simulink model "DFIG_8_asym_voltage_dip_GSC"  (R2022b)
settings: Solver=VariableStepAuto  StartTime=0.0  StopTime=5  RelTol=1e-3
InitFcn:
  | DFIG_init8
values from neighbouring files (symbols this model uses):
  Cbus = 80e-3    (= 0.08)    [DFIG_init4.m]    (also in DFIG_init5.m; DFIG_init6.m; DFIG_init7.m; DFIG_init8.m)
  D = 1e-3    (= 0.001)    [DFIG_init1.m]    (also in DFIG_init3.m; DFIG_init4.m; DFIG_init5.m; DFIG_init6.m)
  f = 50    [DFIG_init1.m]    (also in DFIG_init3.m; DFIG_init4.m; DFIG_init5.m; DFIG_init6.m)
  fsw = 4e3    (= 4000)    [DFIG_init1.m]    (also in DFIG_init3.m; DFIG_init4.m; DFIG_init5.m; DFIG_init6.m)
  Is = 1760    [DFIG_init1.m]    (also in DFIG_init3.m; DFIG_init4.m; DFIG_init5.m; DFIG_init6.m)
  J = 127    [DFIG_init1.m]    (also in DFIG_init3.m = 63.5; DFIG_init4.m = 63.5; DFIG_init5.m; DFIG_init6.m)
  ki_id = (wni^2)*Lr*sigma    (= 491.599501999)    [DFIG_init1.m]    (also in DFIG_init3.m; DFIG_init4.m; DFIG_init5.m; DFIG_init6.m = 19.6639800799)
  ki_idg = (wnig^2)*Lg    (= 56.8489213503)    [DFIG_init4.m]    (also in DFIG_init5.m; DFIG_init6.m; DFIG_init7.m; DFIG_init8.m)
  ki_iq = ki_id    (= 491.599501999)    [DFIG_init1.m]    (also in DFIG_init3.m; DFIG_init4.m; DFIG_init5.m; DFIG_init6.m = 19.6639800799)
  ki_iqg = ki_idg    (= 56.8489213503)    [DFIG_init4.m]    (also in DFIG_init5.m; DFIG_init6.m; DFIG_init7.m; DFIG_init8.m)
  ki_n = (wnn^2)*J/p    (= 25400)    [DFIG_init1.m]    (also in DFIG_init3.m = 12700; DFIG_init4.m = 12700; DFIG_init5.m; DFIG_init6.m)
  ki_v = -300000    [DFIG_init4.m]    (also in DFIG_init5.m; DFIG_init6.m; DFIG_init7.m = -60000; DFIG_init8.m)
  Kopt = ((0.5*ro*pi* (Radio^5) *Cp_max)/(lambda_opt^3))    (= 296454.198186)    [DFIG_init3.m]    (also in DFIG_init4.m; DFIG_init5.m; DFIG_init6.m; DFIG_init7.m)
  kp_id = (2*wni*sigma*Lr)-Rr    (= 0.5771)    [DFIG_init1.m]    (also in DFIG_init3.m; DFIG_init4.m; DFIG_init5.m; DFIG_init6.m = 0.1131)
  kp_idg = (2*wnig*Lg)-Rg    (= 0.301572894745)    [DFIG_init4.m]    (also in DFIG_init5.m; DFIG_init6.m; DFIG_init7.m; DFIG_init8.m)
  kp_iq = kp_id    (= 0.5771)    [DFIG_init1.m]    (also in DFIG_init3.m; DFIG_init4.m; DFIG_init5.m; DFIG_init6.m = 0.1131)
  kp_iqg = kp_idg    (= 0.301572894745)    [DFIG_init4.m]    (also in DFIG_init5.m; DFIG_init6.m; DFIG_init7.m; DFIG_init8.m)
  kp_n = (2*wnn*J)/p    (= 2540)    [DFIG_init1.m]    (also in DFIG_init3.m = 1270; DFIG_init4.m = 1270; DFIG_init5.m; DFIG_init6.m)
  kp_v = -1000    [DFIG_init4.m]    (also in DFIG_init5.m; DFIG_init6.m; DFIG_init7.m; DFIG_init8.m)
  Kpg = 1/(1.5*Vs*sqrt(2/3))    [DFIG_init4.m]    (also in DFIG_init5.m; DFIG_init6.m; DFIG_init7.m; DFIG_init8.m)
  Kqg = -Kpg    [DFIG_init4.m]    (also in DFIG_init5.m; DFIG_init6.m; DFIG_init7.m; DFIG_init8.m)
  kT = -1.5*p*(Lm/Ls)*Fs    [DFIG_init1.m]    (also in DFIG_init3.m; DFIG_init4.m; DFIG_init5.m; DFIG_init6.m)
  Lg = 400e-6    (= 0.0004)    [DFIG_init4.m]    (also in DFIG_init5.m; DFIG_init6.m; DFIG_init7.m; DFIG_init8.m)
  Lr = Lm + Lsi    (= 0.002587)    [DFIG_init1.m]    (also in DFIG_init3.m; DFIG_init4.m; DFIG_init5.m; DFIG_init6.m)
  Lsi = 0.087e-3    (= 8.7e-05)    [DFIG_init1.m]    (also in DFIG_init3.m; DFIG_init4.m; DFIG_init5.m; DFIG_init6.m)
  N = 100    [DFIG_init3.m]    (also in DFIG_init4.m; DFIG_init5.m; DFIG_init6.m; DFIG_init7.m)
  p = 2    [DFIG_init1.m]    (also in DFIG_init3.m; DFIG_init4.m; DFIG_init5.m; DFIG_init6.m)
  Ps = 2e6    (= 2000000)    [DFIG_init1.m]    (also in DFIG_init3.m; DFIG_init4.m; DFIG_init5.m; DFIG_init6.m)
  Radio = 42    [DFIG_init3.m]    (also in DFIG_init4.m; DFIG_init5.m; DFIG_init6.m; DFIG_init7.m)
  Rcrowbar = 0.2    [DFIG_init5.m]    (also in DFIG_init6.m; DFIG_init7.m; DFIG_init8.m; DFIG_init9.m)
  Rg = 20e-6    (= 2e-05)    [DFIG_init4.m]    (also in DFIG_init5.m; DFIG_init6.m; DFIG_init7.m; DFIG_init8.m)
  ro = 1.225    [DFIG_init3.m]    (also in DFIG_init4.m; DFIG_init5.m; DFIG_init6.m; DFIG_init7.m)
  Rr = 2.9e-3    (= 0.0029)    [DFIG_init1.m]    (also in DFIG_init3.m; DFIG_init4.m; DFIG_init5.m; DFIG_init6.m)
  Rs = 2.6e-3    (= 0.0026)    [DFIG_init1.m]    (also in DFIG_init3.m; DFIG_init4.m; DFIG_init5.m; DFIG_init6.m)
  sigma = 1-Lm^2/(Ls*Lr)    (= 0.0661284179513)    [DFIG_init1.m]    (also in DFIG_init3.m; DFIG_init4.m; DFIG_init5.m; DFIG_init6.m)
  smax = 1/3    (= 0.333333333333)    [DFIG_init1.m]    (also in DFIG_init3.m; DFIG_init4.m; DFIG_init5.m; DFIG_init6.m)
  t_dip = 3    [DFIG_init5.m]    (also in DFIG_init6.m = 30; DFIG_init7.m; DFIG_init8.m; DFIG_init9.m)
  t_normal = 4.17    [DFIG_init5.m]    (also in DFIG_init6.m = 417; DFIG_init7.m = 4.2; DFIG_init8.m = 4.2; DFIG_init9.m)
  t_recover = 3.5    [DFIG_init5.m]    (also in DFIG_init6.m = 35; DFIG_init7.m; DFIG_init8.m; DFIG_init9.m)
  tab_lambda = [0.1:0.01:11.8]    [DFIG_init3.m]    (also in DFIG_init4.m; DFIG_init5.m; DFIG_init6.m; DFIG_init7.m)
  Tcrowbar = 0.1    [DFIG_init5.m]    (also in DFIG_init6.m; DFIG_init7.m; DFIG_init8.m; DFIG_init9.m)
  Tem = 12732    [DFIG_init1.m]    (also in DFIG_init3.m; DFIG_init4.m; DFIG_init5.m; DFIG_init6.m)
  Ts = 1/fsw/50    (= 5e-06)    [DFIG_init1.m]    (also in DFIG_init3.m; DFIG_init4.m; DFIG_init5.m; DFIG_init6.m)
  Vbus = Vr_stator*sqrt(2)    [DFIG_init1.m]    (also in DFIG_init3.m; DFIG_init4.m = 1150; DFIG_init5.m = 1150; DFIG_init6.m = 1150)
  Vs = 690    [DFIG_init1.m]    (also in DFIG_init3.m; DFIG_init4.m; DFIG_init5.m; DFIG_init6.m)
undefined symbols (not defined in the file or in its folder): Ct, DiscIntNeverNeededParam
libraries: spsSeriesRLCBranchLib x5, spsSecondOrderFilterLib x4, spsUniversalBridgeLib x3, spsThreePhaseVIMeasurementLib x3, spsPLL3phLib x2, spsPWMGenerator2LevelLib x2, spsAsynchronousMachineSIUnitsLib x1, spsGroundLib x1, spsIdealSwitchLib x1, spsThreePhaseProgrammableVoltageSourceLib x1, spsThreePhaseTransformerTwoWindingsLib x1, spsEdgeDetectorLib x1
settings Model: SimulationMode=accelerator  Creator=Qingyuan  LastModifiedBy=Qingyuan

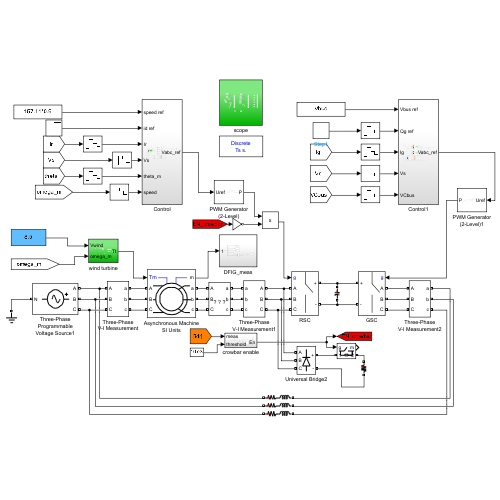
[thumbnail: Simulink's stored preview of the top-level diagram]
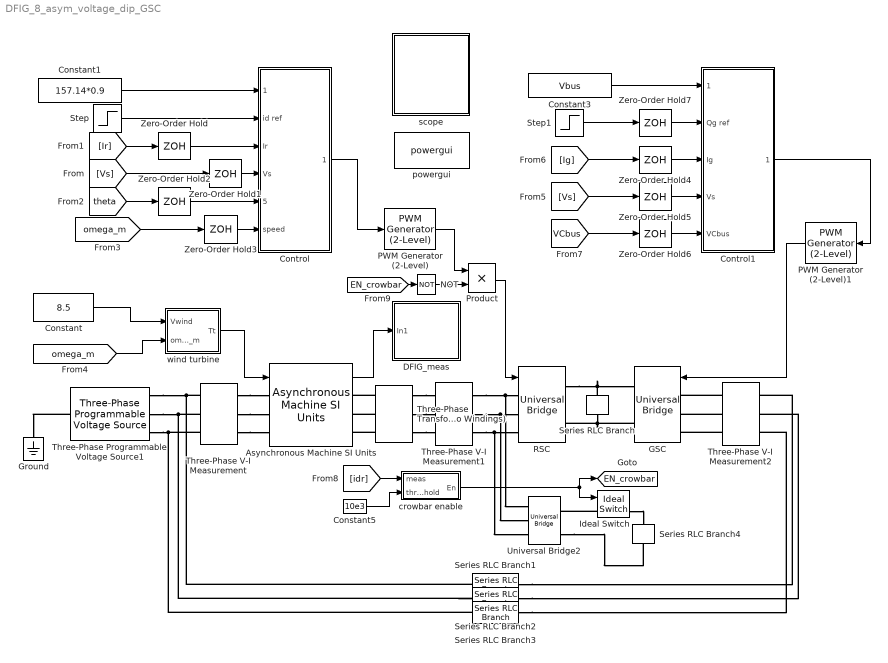
== system DFIG_8_asym_voltage_dip_GSC ==
  Asynchronous Machine SI Units : spsAsynchronousMachineSIUnitsLib/Asynchronous Machine SI Units  RotorType=Wound  PresetModel=No  MechanicalLoad=Torque Tm  ShowDetailedParameters=on  ReferenceFrame=Rotor  Units=SI  MeasurementBus=off  NominalParameters=[Ps Vs f]  VoltageRatio=1  Stator=[Rs Lsi]  Rotor=[Rr Lsi]  Cage1=[0.4155 0.002066]  Cage2=[0.4168 0.0003495]  Lm=Lm  Mechanical=[J D p]  PolePairs=2  InitialConditions=[1 0 0 0 0 0 0 0]  SimulateSaturation=off  Saturation=[14.03593122, 27.81365428, 53.79336849, 72.68890987, 97.98006896, 148.6815601, 215.7428561, 302.9841135, 428.7778367 ; 230, 322, 414, 460, 506, 552, 598, 644, 690]  LoadFlowParameters=1492000  TsPowergui=0  TsBlock=-1  IterativeModel=Trapezoidal non iterative  IterativeDiscreteModel=Trapezoidal non iterative  Pmec=1.4e6
  Constant : Constant  Value=8.5
  Constant1 : Constant  Value=157.14*0.9
  Constant3 : Constant  Value=Vbus
  Constant5 : Constant  Value=10e3
  Control : Subsystem
  Control1 : Subsystem
  DFIG_meas : Subsystem
  GSC : spsUniversalBridgeLib/Universal Bridge  Arms=3  SnubberResistance=1e5  SnubberCapacitance=inf  Device=Ideal Switches  Ron=1e-3  Lon=0  ForwardVoltages="[  0  0  ]"  ForwardVoltage=0  GTOparameters=[ 10e-6 , 20e-6 ]  IGBTparameters=[ 1e-6 , 2e-6 ]  Measurements=None  Measurements_2=None  converterType=Rectifier
  Ground : spsGroundLib/Ground  LConnTagsString=a
  Ideal Switch : spsIdealSwitchLib/Ideal Switch  Ron=0.001  Lon=0  IC=0  Rs=1e5  Cs=inf  Measurements=on
  NOT : Logic  Operator=NOT  IconShape=distinctive  AllPortsSameDT=off  OutDataTypeStr=boolean
  PWM Generator (2-Level) : spsPWMGenerator2LevelLib/PWM Generator (2-Level)  ModulatorType=Three-phase bridge (6 pulses)  ModulatorMode=Unsynchronized  Fc=fsw  Pc=0  nF=27  MinMax="[ -1  1 ]"  SamplingTechnique=Symmetrical regular (single edge)  ModulatingSignals=off  m=0.8  Freq=60  Phase=0  Ts=0  ShowCarrierOutport=off
  PWM Generator (2-Level)1 : spsPWMGenerator2LevelLib/PWM Generator (2-Level)  ModulatorType=Three-phase bridge (6 pulses)  ModulatorMode=Unsynchronized  Fc=fsw  Pc=0  nF=27  MinMax="[ -1  1 ]"  SamplingTechnique=Symmetrical regular (single edge)  ModulatingSignals=off  m=0.8  Freq=60  Phase=0  Ts=0  ShowCarrierOutport=off
  Product : Product
  RSC : spsUniversalBridgeLib/Universal Bridge  Arms=3  SnubberResistance=1e5  SnubberCapacitance=inf  Device=Ideal Switches  Ron=1e-3  Lon=0  ForwardVoltages="[  0  0  ]"  ForwardVoltage=0  GTOparameters=[ 10e-6 , 20e-6 ]  IGBTparameters=[ 1e-6 , 2e-6 ]  Measurements=None  Measurements_2=None  converterType=Rectifier
  Series RLC Branch : spsSeriesRLCBranchLib/Series RLC Branch  LConnTagsString=__new0  RConnTagsString=__new0  BranchType=C  Resistance=1  Inductance=1e-3  SetiL0=off  InitialCurrent=0  Capacitance=Cbus  Setx0=off  InitialVoltage=0  Measurements=Branch voltage
  Series RLC Branch1 : spsSeriesRLCBranchLib/Series RLC Branch  LConnTagsString=__new0  RConnTagsString=__new0  BranchType=RL  Resistance=Rg  Inductance=Lg  SetiL0=off  InitialCurrent=0  Capacitance=1e-6  Setx0=off  InitialVoltage=0  Measurements=None
  Series RLC Branch2 : spsSeriesRLCBranchLib/Series RLC Branch  LConnTagsString=__new0  RConnTagsString=__new0  BranchType=RL  Resistance=Rg  Inductance=Lg  SetiL0=off  InitialCurrent=0  Capacitance=1e-6  Setx0=off  InitialVoltage=0  Measurements=None
  Series RLC Branch3 : spsSeriesRLCBranchLib/Series RLC Branch  LConnTagsString=__new0  RConnTagsString=__new0  BranchType=RL  Resistance=Rg  Inductance=Lg  SetiL0=off  InitialCurrent=0  Capacitance=1e-6  Setx0=off  InitialVoltage=0  Measurements=None
  Series RLC Branch4 : spsSeriesRLCBranchLib/Series RLC Branch  LConnTagsString=__new0  RConnTagsString=__new0  BranchType=R  Resistance=Rcrowbar  Inductance=1e-3  SetiL0=off  InitialCurrent=0  Capacitance=Cbus  Setx0=off  InitialVoltage=0  Measurements=Branch current
  Step : Step  Time=t_dip+0.1  After=0.25*Is  SampleTime=0
  Step1 : Step  Time=t_dip+0.1  After=-500e3  SampleTime=0
  Three-Phase Programmable Voltage Source1 : spsThreePhaseProgrammableVoltageSourceLib/Three-Phase Programmable Voltage Source  PositiveSequence=[Vs 0 f]  VariationEntity=None  VariationType=Ramp  VariationTypeAlt=Step  VariationStep=0.5  VariationRate=15  VariationMagnitude=0.3  VariationFrequency=2  VariationTiming=[t_recover t_normal]  VariationPhaseA=off  Amplitudes=[1 0.8 1.2 1.0]  TimeValues=[0 0.1 0.15 0.2]  HarmonicGeneration=on  HarmonicA=[1 0.3 180 1]  HarmonicB=[1 0.2 0 2]  Timing="[t_dip  t_normal]"  BusType=swing  Pref=0  Qref=0  Qmin=-inf  Qmax=inf
  Three-Phase Transformer (Two Windings) : spsThreePhaseTransformerTwoWindingsLib/Three-Phase Transformer (Two Windings)  Winding1Connection=Y  Winding2Connection=Y  CoreType=Three single-phase transformers  SetSaturation=off  Hysteresis=off  DataFile='hysteresis'  SetInitialFlux=off  Measurements=None  UNITS=SI  NominalPower=[ Ps , f ]  Winding1=[Vs 0 0]  Winding2=[Vs/u 0 0]  Rm=1.3506e+08  Lm=4.299e+05  L0=0.5  Saturation=[0 0;0.0053322 2292.3;2.2218 2903.6]  InitialFluxes=[ 0.8 , -0.8 , 0.7 ]  BreakLoop=off  DiscreteSolver=Trapezoidal iterative  DataType=on  TransfoNumber=1
  Three-Phase V-I Measurement : spsThreePhaseVIMeasurementLib/Three-Phase V-I Measurement  VoltageMeasurement=phase-to-ground  SetLabelV=on  LabelV=Vs  Vpu=off  VpuLL=off  CurrentMeasurement=yes  SetLabelI=on  LabelI=Is  Ipu=off  Pbase=100e6  Vbase=500e3  OutputType=Complex  PhasorSimulation=off  PSBequivalent=0
  Three-Phase V-I Measurement1 : spsThreePhaseVIMeasurementLib/Three-Phase V-I Measurement  VoltageMeasurement=no  SetLabelV=off  LabelV=Vc  Vpu=off  VpuLL=off  CurrentMeasurement=yes  SetLabelI=on  LabelI=Ir  Ipu=off  Pbase=100e6  Vbase=500e3  OutputType=Complex  PhasorSimulation=off  PSBequivalent=0
  Three-Phase V-I Measurement2 : spsThreePhaseVIMeasurementLib/Three-Phase V-I Measurement  VoltageMeasurement=no  SetLabelV=off  LabelV=Vc  Vpu=off  VpuLL=off  CurrentMeasurement=yes  SetLabelI=on  LabelI=Ig  Ipu=off  Pbase=100e6  Vbase=500e3  OutputType=Complex  PhasorSimulation=off  PSBequivalent=0
  Universal Bridge2 : spsUniversalBridgeLib/Universal Bridge  Arms=3  SnubberResistance=1e5  SnubberCapacitance=inf  Device=Diodes  Ron=1e-3  Lon=0  ForwardVoltages="[  0  0  ]"  ForwardVoltage=0  GTOparameters=[ 10e-6 , 20e-6 ]  IGBTparameters=[ 1e-6 , 2e-6 ]  Measurements=None  Measurements_2=None  converterType=Rectifier
  Zero-Order Hold{,1..7} (8 alike) : ZeroOrderHold  SampleTime=1/fsw
  crowbar enable : Subsystem
  powergui : spspowerguiLib/powergui  Priority=1  SimulationMode=Discrete  SampleTime=Ts  frequency=60  Iterations=50  frequencyindice=50  Pbase=100e6  ErrMax=1e-4  UnitsV=kV  UnitsW=MW  buscounter=0  FunctionMessages=off  echomessages=off  EnableUseOfTLC=off  CurrentSourceSwitches=off  DisableSnubberDevices=off  DisableRonSwitches=off  DisableVfSwitches=off  DisplayEquations=off  AutomaticDiscreteSolvers=off  SolverType=Tustin/Backward Euler (TBE)  Interpol=off  ExternalGateDelay=off  methode=off  Ts=100  x0status=blocks  SPID=on  SwTol=0  HookPort=off  NonlinearTolerance=1e-4  nMaxIteration=100  ContinueOnMaxIteration=off  RestoreLinks=warning  ResistiveCurrentMeasurement=off  Frange=[0:2:500]  Ylog=off  Xlog=on  ShowGrid=off  save=off  variable=ZData  structure=0  ZoomFFT=off  StartTime=0.0  cycles=1  DisplayStyle=1  fundamental=60  FreqAxis=off  MaxFrequency=1000  frequencyindicesteady=1  RmsSteady=1  display=off
  scope : Subsystem
  wind turbine : Subsystem
  tag scope: EN_crowbar=global
  wires:
  Control/1(Vabc_ref) -> PWM Generator (2-Level)/1
  [Vs] -> Zero-Order Hold1/1
  [Ir] -> Zero-Order Hold/1
  Constant1/1 -> Control/1(speed ref)
  Step/1 -> Control/2(id ref)
  [theta] -> Zero-Order Hold2/1
  [omega_m] -> Zero-Order Hold3/1
  Asynchronous Machine SI Units/1 -> DFIG_meas/1(In1)
  Zero-Order Hold/1 -> Control/3(Ir)
  Zero-Order Hold1/1 -> Control/4(Vs)
  Zero-Order Hold2/1 -> Control/5(theta_m)
  Zero-Order Hold3/1 -> Control/6(speed)
  Constant/1 -> wind turbine/1(Vwind)
  wind turbine/1(Tt) -> Asynchronous Machine SI Units/1
  [omega_m] -> wind turbine/2(omega_m)
  Zero-Order Hold5/1 -> Control1/4(Vs)
  Zero-Order Hold4/1 -> Control1/3(Ig)
  Constant3/1 -> Control1/1(Vbus ref)
  [Ig] -> Zero-Order Hold4/1
  [Vs] -> Zero-Order Hold5/1
  Control1/1(Vabc_ref) -> PWM Generator (2-Level)1/1
  [VCbus] -> Zero-Order Hold6/1
  Zero-Order Hold6/1 -> Control1/5(VCbus)
  Zero-Order Hold7/1 -> Control1/2(Qg ref)
  Constant5/1 -> crowbar enable/2(threshold)
  crowbar enable/1(En) -> Ideal Switch/1, [EN_crowbar]
  [idr] -> crowbar enable/1(meas)
  NOT/1 -> Product/2
  [EN_crowbar] -> NOT/1
  PWM Generator (2-Level)1/1 -> GSC/1
  PWM Generator (2-Level)/1 -> Product/1
  Product/1 -> RSC/1
  Step1/1 -> Zero-Order Hold7/1
  connections:
  Three-Phase Programmable Voltage Source1/LConn1 -- Ground/LConn1
  Three-Phase V-I Measurement/LConn1 -- Three-Phase Programmable Voltage Source1/RConn1 -- Series RLC Branch1/LConn1
  Three-Phase V-I Measurement/LConn2 -- Three-Phase Programmable Voltage Source1/RConn2 -- Series RLC Branch2/LConn1
  Three-Phase V-I Measurement/LConn3 -- Series RLC Branch3/LConn1 -- Three-Phase Programmable Voltage Source1/RConn3
  Three-Phase V-I Measurement/RConn1 -- Asynchronous Machine SI Units/LConn1
  Three-Phase V-I Measurement/RConn2 -- Asynchronous Machine SI Units/LConn2
  Three-Phase V-I Measurement/RConn3 -- Asynchronous Machine SI Units/LConn3
  Three-Phase V-I Measurement1/LConn1 -- Universal Bridge2/LConn1 -- RSC/LConn1
  Three-Phase V-I Measurement1/LConn3 -- Universal Bridge2/LConn3 -- RSC/LConn3
  Three-Phase V-I Measurement1/LConn2 -- Universal Bridge2/LConn2 -- RSC/LConn2
  Three-Phase Transformer (Two Windings)/RConn1 -- Three-Phase V-I Measurement1/RConn1
  Three-Phase Transformer (Two Windings)/RConn2 -- Three-Phase V-I Measurement1/RConn2
  Three-Phase Transformer (Two Windings)/RConn3 -- Three-Phase V-I Measurement1/RConn3
  RSC/RConn1 -- Series RLC Branch/LConn1 -- GSC/RConn1
  GSC/RConn2 -- RSC/RConn2 -- Series RLC Branch/RConn1
  Three-Phase V-I Measurement2/LConn1 -- GSC/LConn1
  Three-Phase V-I Measurement2/LConn2 -- GSC/LConn2
  Three-Phase V-I Measurement2/LConn3 -- GSC/LConn3
  Series RLC Branch1/RConn1 -- Three-Phase V-I Measurement2/RConn1
  Series RLC Branch2/RConn1 -- Three-Phase V-I Measurement2/RConn2
  Series RLC Branch3/RConn1 -- Three-Phase V-I Measurement2/RConn3
  Three-Phase Transformer (Two Windings)/LConn3 -- Asynchronous Machine SI Units/RConn3
  Three-Phase Transformer (Two Windings)/LConn2 -- Asynchronous Machine SI Units/RConn2
  Three-Phase Transformer (Two Windings)/LConn1 -- Asynchronous Machine SI Units/RConn1
  Ideal Switch/LConn1 -- Universal Bridge2/RConn1
  Ideal Switch/RConn1 -- Series RLC Branch4/LConn1
  Universal Bridge2/RConn2 -- Series RLC Branch4/RConn1

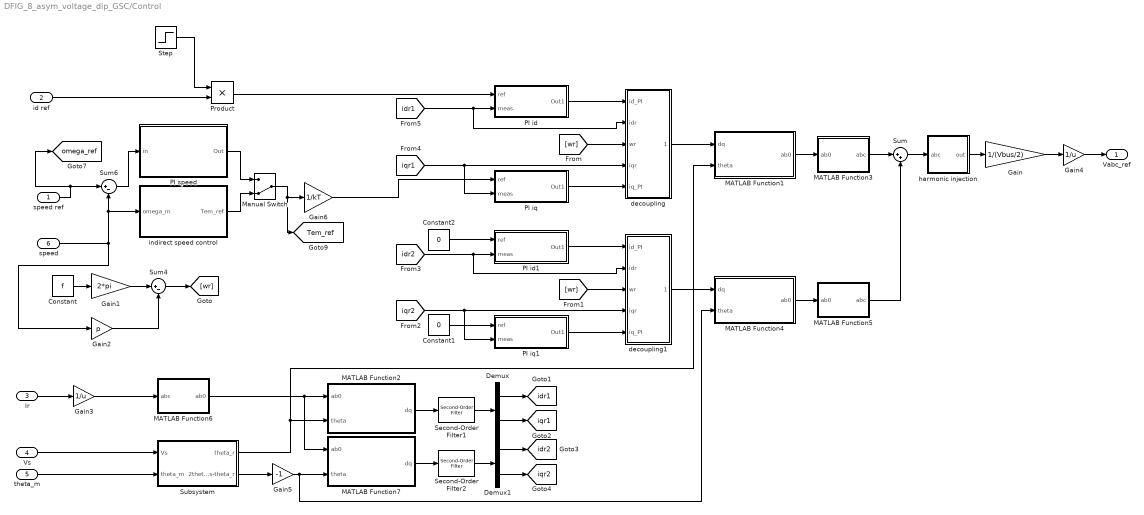
== system DFIG_8_asym_voltage_dip_GSC/Control ==
  speed ref : Inport
  id ref : Inport  Port=2
  Ir : Inport  Port=3
  Vs : Inport  Port=4
  theta_m : Inport  Port=5
  speed : Inport  Port=6
  Constant : Constant  Value=f
  Constant1 : Constant  Value=0
  Constant2 : Constant  Value=0
  Demux : Demux  Outputs=2
  Demux1 : Demux  Outputs=2
  Gain : Gain  Gain=1/(Vbus/2)
  Gain1 : Gain  Gain=2*pi
  Gain2 : Gain  Gain=p
  Gain3 : Gain  Gain=1/u
  Gain4 : Gain  Gain=1/u
  Gain5 : Gain  Gain=-1
  Gain6 : Gain  Gain=1/kT
  MATLAB Function1 : MATLAB Function  TreatAsAtomicUnit=on
  MATLAB Function2 : MATLAB Function  TreatAsAtomicUnit=on
  MATLAB Function3 : MATLAB Function  TreatAsAtomicUnit=on
  MATLAB Function4 : MATLAB Function  TreatAsAtomicUnit=on
  MATLAB Function5 : MATLAB Function  TreatAsAtomicUnit=on
  MATLAB Function6 : MATLAB Function  TreatAsAtomicUnit=on
  MATLAB Function7 : MATLAB Function  TreatAsAtomicUnit=on
  Manual Switch : ManualSwitch  CurrentSetting=0
  PI id : Subsystem
  PI id1 : Subsystem
  PI iq : Subsystem
  PI iq1 : Subsystem
  PI speed : Subsystem
  Product : Product
  Second-Order Filter1 : spsSecondOrderFilterLib/Second-Order Filter  FilterType=Bandstop (Notch)  Fo=100  Zeta=0.707  Ts=0  Initialize=on  Vac_Init="[0,  0,  50]"  Vdc_Init=0  PlotResponse=off  FreqRange=[0, 500, 1]
      settings: LibrarySourceBlock=|
      | sps_lib/Control/Filters/Second-Order
      | Filter
  Second-Order Filter2 : spsSecondOrderFilterLib/Second-Order Filter  FilterType=Bandstop (Notch)  Fo=100  Zeta=0.707  Ts=0  Initialize=on  Vac_Init="[0,  0,  50]"  Vdc_Init=0  PlotResponse=off  FreqRange=[0, 500, 1]
      settings: LibrarySourceBlock=|
      | sps_lib/Control/Filters/Second-Order
      | Filter
  Step : Step  Time=t_normal+1  Before=1  After=0  SampleTime=0
  Subsystem : Subsystem
  Sum : Sum  Inputs=|++
  Sum4 : Sum  Inputs=|+-
  Sum6 : Sum  Inputs=|+-
  decoupling : Subsystem
  decoupling1 : Subsystem
  harmonic injection : Subsystem
  indirect speed control : Subsystem
  Vabc_ref : Outport
  tag scope: Tem_ref=global, idr1=global, idr2=global, iqr1=global, iqr2=global, omega_ref=global
  wires:
  MATLAB Function1/1(ab0) -> MATLAB Function3/1(ab0)
  Gain/1 -> Gain4/1
  harmonic injection/1(out) -> Gain/1
  Vs/1 -> Subsystem/1(Vs)
  theta_m/1 -> Subsystem/2(theta_m)
  MATLAB Function6/1(ab0) -> MATLAB Function7/1(ab0), MATLAB Function2/1(ab0)
  Ir/1 -> Gain3/1
  Subsystem/1(theta_r) -> MATLAB Function2/2(theta), MATLAB Function1/2(theta)
  Constant/1 -> Gain1/1
  Gain1/1 -> Sum4/1
  Gain2/1 -> Sum4/2
  Sum4/1 -> [wr]
  MATLAB Function2/1(dq) -> Second-Order Filter1/1
  Demux/2 -> [iqr1]
  Demux/1 -> [idr1]
  Sum6/1 -> PI speed/1(in)
  speed ref/1 -> [omega_ref], Sum6/1
  [idr1] -> decoupling/2(idr), PI id/2(meas)
  [iqr1] -> PI iq/2(meas), decoupling/4(iqr)
  Manual Switch/1 -> [Tem_ref], Gain6/1
  PI speed/1(Out) -> Manual Switch/1
  indirect speed control/1(Tem_ref) -> Manual Switch/2
  speed/1 -> Gain2/1, indirect speed control/1(omega_m), Sum6/2
  Gain3/1 -> MATLAB Function6/1(abc)
  Gain4/1 -> Vabc_ref/1
  id ref/1 -> Product/2
  Step/1 -> Product/1
  [wr] -> decoupling/3(wr)
  decoupling/1(Vref_dq) -> MATLAB Function1/1(dq)
  Product/1 -> PI id/1(ref)
  PI id/1(Out1) -> decoupling/1(id_PI)
  Gain6/1 -> PI iq/1(ref)
  PI iq/1(Out1) -> decoupling/5(iq_PI)
  PI iq1/1(Out1) -> decoupling1/5(iq_PI)
  PI id1/1(Out1) -> decoupling1/1(id_PI)
  decoupling1/1(Vref_dq) -> MATLAB Function4/1(dq)
  [wr] -> decoupling1/3(wr)
  [iqr2] -> decoupling1/4(iqr), PI iq1/2(meas)
  [idr2] -> PI id1/2(meas), decoupling1/2(idr)
  MATLAB Function4/1(ab0) -> MATLAB Function5/1(ab0)
  Constant1/1 -> PI iq1/1(ref)
  Constant2/1 -> PI id1/1(ref)
  MATLAB Function3/1(abc) -> Sum/1
  Sum/1 -> harmonic injection/1(abc)
  MATLAB Function5/1(abc) -> Sum/2
  Subsystem/2(2theta_s-theta_r) -> Gain5/1
  Gain5/1 -> MATLAB Function4/2(theta), MATLAB Function7/2(theta)
  Demux1/1 -> [idr2]
  Demux1/2 -> [iqr2]
  MATLAB Function7/1(dq) -> Second-Order Filter2/1
  Second-Order Filter1/1 -> Demux/1
  Second-Order Filter2/1 -> Demux1/1

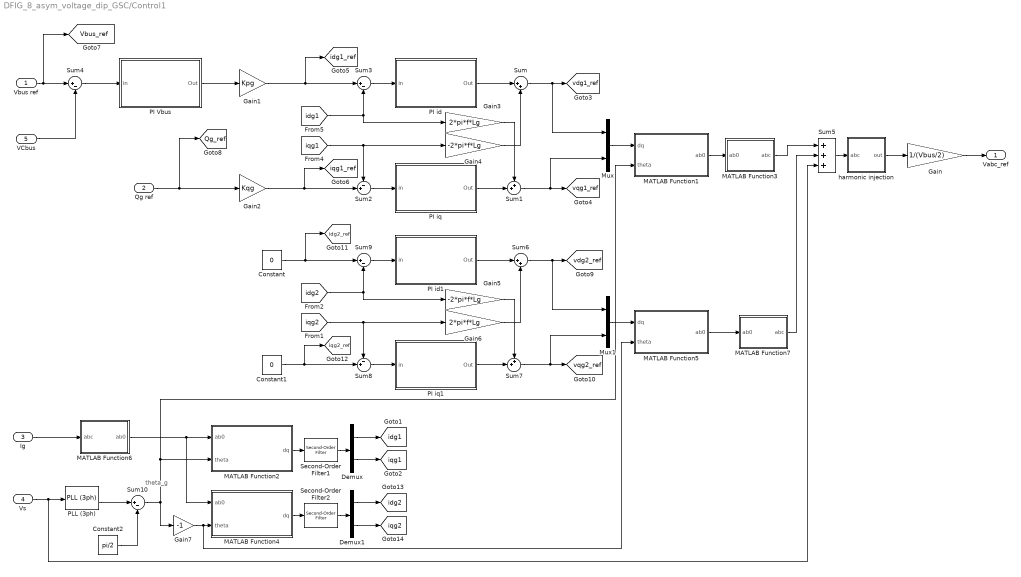
== system DFIG_8_asym_voltage_dip_GSC/Control1 ==
  note: theta_g
  Vbus ref : Inport
  Qg ref : Inport  Port=2
  Ig : Inport  Port=3
  Vs : Inport  Port=4
  VCbus : Inport  Port=5
  Constant : Constant  Value=0
  Constant1 : Constant  Value=0
  Constant2 : Constant  Value=pi/2
  Demux : Demux  Outputs=2
  Demux1 : Demux  Outputs=2
  Gain : Gain  Gain=1/(Vbus/2)
  Gain1 : Gain  Gain=Kpg
  Gain2 : Gain  Gain=Kqg
  Gain3 : Gain  Gain=2*pi*f*Lg
  Gain4 : Gain  Gain=-2*pi*f*Lg
  Gain5 : Gain  Gain=-2*pi*f*Lg
  Gain6 : Gain  Gain=2*pi*f*Lg
  Gain7 : Gain  Gain=-1
  MATLAB Function1 : MATLAB Function  TreatAsAtomicUnit=on
  MATLAB Function2 : MATLAB Function  TreatAsAtomicUnit=on
  MATLAB Function3 : MATLAB Function  TreatAsAtomicUnit=on
  MATLAB Function4 : MATLAB Function  TreatAsAtomicUnit=on
  MATLAB Function5 : MATLAB Function  TreatAsAtomicUnit=on
  MATLAB Function6 : MATLAB Function  TreatAsAtomicUnit=on
  MATLAB Function7 : MATLAB Function  TreatAsAtomicUnit=on
  Mux : Mux  Inputs=2
  Mux1 : Mux  Inputs=2
  PI Vbus : Subsystem
  PI id : Subsystem
  PI id1 : Subsystem
  PI iq : Subsystem
  PI iq1 : Subsystem
  PLL (3ph) : spsPLL3phLib/PLL (3ph)  Fmin=45  Par_Init=[0, 50]  ParK=[180, 3200, 1]  TcD=0.01  MaxRateChangeFreq=12  FilterCutOffFreq=25  Ts=1/fsw  AGC=on
  Second-Order Filter1 : spsSecondOrderFilterLib/Second-Order Filter  FilterType=Bandstop (Notch)  Fo=100  Zeta=0.707  Ts=0  Initialize=on  Vac_Init="[0,  0,  50]"  Vdc_Init=0  PlotResponse=off  FreqRange=[0, 500, 1]
      settings: LibrarySourceBlock=|
      | sps_lib/Control/Filters/Second-Order
      | Filter
  Second-Order Filter2 : spsSecondOrderFilterLib/Second-Order Filter  FilterType=Bandstop (Notch)  Fo=100  Zeta=0.707  Ts=0  Initialize=on  Vac_Init="[0,  0,  50]"  Vdc_Init=0  PlotResponse=off  FreqRange=[0, 500, 1]
      settings: LibrarySourceBlock=|
      | sps_lib/Control/Filters/Second-Order
      | Filter
  Sum : Sum  Inputs=|++
  Sum1 : Sum  Inputs=++|
  Sum{3..4,9..10} (4 alike) : Sum  Inputs=|+-
  Sum2 : Sum  Inputs=-+|
  Sum5 : Sum  Inputs=+++
  Sum6 : Sum  Inputs=|++
  Sum7 : Sum  Inputs=++|
  Sum8 : Sum  Inputs=-+|
  harmonic injection : Subsystem
  Vabc_ref : Outport
  tag scope: Qg_ref=global, Vbus_ref=global, idg1=global, idg1_ref=global, idg2=global, idg2_ref=global, iqg1=global, iqg1_ref=global, iqg2=global, iqg2_ref=global, vdg1_ref=global, vdg2_ref=global, vqg1_ref=global, vqg2_ref=global
  wires:
  PI Vbus/1(Out) -> Gain1/1
  [iqg1] -> Sum2/1, Gain4/1
  Gain3/1 -> Sum1/1
  PI iq/1(Out) -> Sum1/2
  Gain4/1 -> Sum/2
  PI id/1(Out) -> Sum/1
  [idg1] -> Gain3/1, Sum3/2
  Gain2/1 -> Sum2/2, [iqg1_ref]
  Mux/1 -> MATLAB Function1/1(dq)
  Sum1/1 -> Mux/2, [vqg1_ref]
  Sum/1 -> [vdg1_ref], Mux/1
  Demux/1 -> [idg1]
  Demux/2 -> [iqg1]
  MATLAB Function2/1(dq) -> Second-Order Filter1/1
  Sum3/1 -> PI id/1(in)
  Sum2/1 -> PI iq/1(in)
  Ig/1 -> MATLAB Function6/1(abc)
  MATLAB Function6/1(ab0) -> MATLAB Function4/1(ab0), MATLAB Function2/1(ab0)
  harmonic injection/1(out) -> Gain/1
  Gain/1 -> Vabc_ref/1
  MATLAB Function1/1(ab0) -> MATLAB Function3/1(ab0)
  Gain1/1 -> [idg1_ref], Sum3/1
  Qg ref/1 -> [Qg_ref], Gain2/1
  VCbus/1 -> Sum4/2
  Vbus ref/1 -> [Vbus_ref], Sum4/1
  Sum4/1 -> PI Vbus/1(in)
  Sum5/1 -> harmonic injection/1(abc)
  MATLAB Function3/1(abc) -> Sum5/1
  Constant/1 -> [idg2_ref], Sum9/1
  MATLAB Function5/1(ab0) -> MATLAB Function7/1(ab0)
  Sum8/1 -> PI iq1/1(in)
  Sum9/1 -> PI id1/1(in)
  Sum6/1 -> Mux1/1, [vdg2_ref]
  Sum7/1 -> [vqg2_ref], Mux1/2
  Mux1/1 -> MATLAB Function5/1(dq)
  Constant1/1 -> [iqg2_ref], Sum8/2
  [idg2] -> Sum9/2, Gain5/1
  PI id1/1(Out) -> Sum6/1
  Gain6/1 -> Sum6/2
  PI iq1/1(Out) -> Sum7/2
  Gain5/1 -> Sum7/1
  [iqg2] -> Gain6/1, Sum8/1
  Constant2/1 -> Sum10/2
  PLL (3ph)/2 -> Sum10/1
  Vs/1 -> Sum5/3, PLL (3ph)/1
  Second-Order Filter1/1 -> Demux/1
  Sum10/1 -> Gain7/1, MATLAB Function2/2(theta), MATLAB Function1/2(theta)
  Second-Order Filter2/1 -> Demux1/1
  MATLAB Function4/1(dq) -> Second-Order Filter2/1
  Demux1/2 -> [iqg2]
  Demux1/1 -> [idg2]
  Gain7/1 -> MATLAB Function5/2(theta), MATLAB Function4/2(theta)
  MATLAB Function7/1(abc) -> Sum5/2

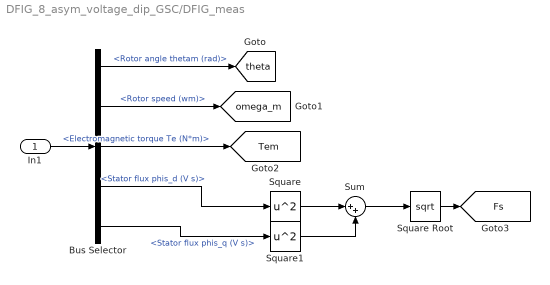
== system DFIG_8_asym_voltage_dip_GSC/DFIG_meas ==
  In1 : Inport
  Bus Selector : BusSelector  OutputSignals=Mechanical.Rotor angle thetam (rad),Mechanical.Rotor speed (wm),Mechanical.Electromagnetic torque Te (N*m),Stator measurements.Stator flux phis_d (V s),Stator measurements.Stator flux phis_q (V s)
  Square : Math  Operator=square
  Square Root : Sqrt
  Square1 : Math  Operator=square
  Sum : Sum  Inputs=|++
  tag scope: Fs=global, Tem=global, omega_m=global, theta=global
  wires:
  Bus Selector/1 -> [theta]  "<Rotor angle thetam (rad)>"
  Bus Selector/2 -> [omega_m]  "<Rotor speed (wm)>"
  In1/1 -> Bus Selector/1
  Bus Selector/3 -> [Tem]  "<Electromagnetic torque Te (N*m)>"
  Bus Selector/4 -> Square/1  "<Stator flux phis_d (V s)>"
  Bus Selector/5 -> Square1/1  "<Stator flux phis_q (V s)>"
  Square/1 -> Sum/1
  Sum/1 -> Square Root/1
  Square1/1 -> Sum/2
  Square Root/1 -> [Fs]

== system DFIG_8_asym_voltage_dip_GSC/crowbar enable ==
  meas : Inport
  threshold : Inport  Port=2
  Delay : Delay  DelayLength=Tcrowbar*fsw  SampleTime=1/fsw
  Edge Detector : spsEdgeDetectorLib/Edge Detector  model=Rising  ic=0  Ts=1/fsw
      settings: LibrarySourceBlock=sps_lib/Control/Edge Detector
  Relational Operator : RelationalOperator  OutDataTypeStr=boolean  RndMeth=Simplest  InputSameDT=off
  Scope : Scope  NumInputPorts=3
  Set-Reset Flip-Flop : eeGeneralControl/Set-Reset Flip-Flop  LabelModeActiveChoice=Discrete  UndefState=Set  Q0=0  Ts=0.5/fsw
      settings: LibrarySourceBlock=ee_sl_lib/General Control/Set-Reset Flip-Flop
  En : Outport
  wires:
  threshold/1 -> Relational Operator/2
  Relational Operator/1 -> Edge Detector/1
  meas/1 -> Scope/1, Relational Operator/1
  Edge Detector/1 -> Delay/1, Set-Reset Flip-Flop/1, Scope/2
  Delay/1 -> Set-Reset Flip-Flop/2
  Set-Reset Flip-Flop/1 -> En/1, Scope/3

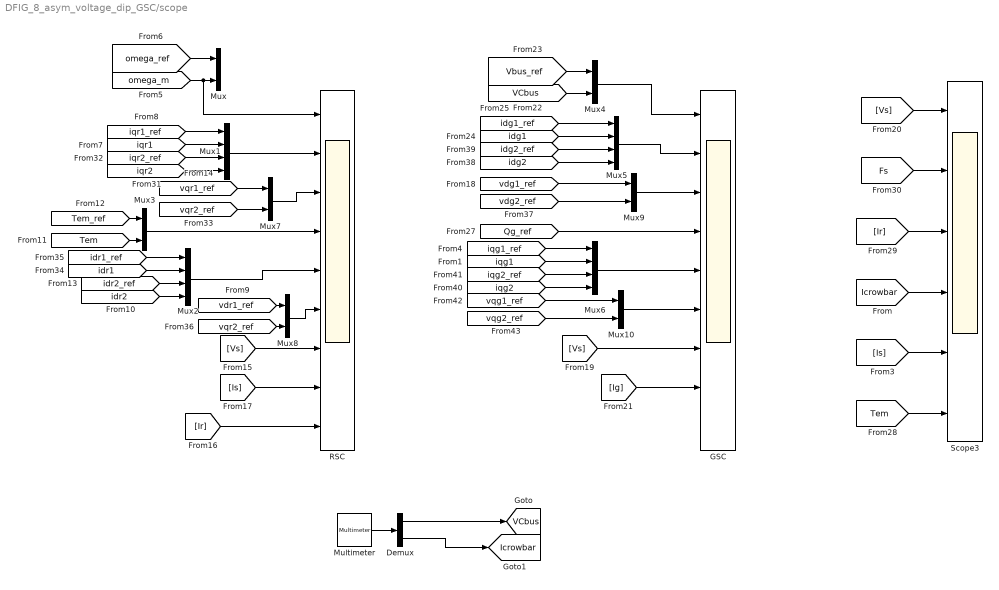
== system DFIG_8_asym_voltage_dip_GSC/scope ==
  Demux : Demux  Outputs=2
  GSC : Scope  NumInputPorts=9
  Multimeter : spsMultimeterLib/Multimeter  L=2  sel=[1 2]  yselected={}  Gain=[1 1]  OutputType=Complex  PlotAtSimulationStop=off  PhasorSimulation=off
  Mux{,3..4,7..10} (7 alike) : Mux  Inputs=2
  Mux{1..2,5..6} (4 alike) : Mux
  RSC : Scope  NumInputPorts=9
  Scope3 : Scope  NumInputPorts=6
  tag scope: Icrowbar=global, VCbus=global
  wires:
  [omega_ref] -> Mux/1
  [iqr1] -> Mux1/2
  [omega_m] -> RSC/1, Mux/2
  [Vs] -> RSC/7
  [Tem] -> Mux3/2
  [Ir] -> RSC/9
  [Tem_ref] -> Mux3/1
  Mux1/1 -> RSC/2
  [vqr1_ref] -> Mux7/1
  Mux3/1 -> RSC/4
  [iqr1_ref] -> Mux1/1
  [Is] -> RSC/8
  [Ig] -> GSC/8
  Mux6/1 -> GSC/5
  [idg1_ref] -> Mux5/1
  [iqg1_ref] -> Mux6/1
  [vdg1_ref] -> Mux9/1
  [iqg1] -> Mux6/2
  Mux5/1 -> GSC/2
  [Vs] -> GSC/7
  [VCbus] -> Mux4/2
  [idg1] -> Mux5/2
  [Vbus_ref] -> Mux4/1
  Mux4/1 -> GSC/1
  [Qg_ref] -> GSC/4
  Multimeter/1 -> Demux/1
  Demux/1 -> [VCbus]
  Demux/2 -> [Icrowbar]
  [Icrowbar] -> Scope3/4
  [Vs] -> Scope3/1
  [Is] -> Scope3/5
  [Tem] -> Scope3/6
  [Ir] -> Scope3/3
  [Fs] -> Scope3/2
  [iqr2_ref] -> Mux1/3
  [iqr2] -> Mux1/4
  [vqr2_ref] -> Mux7/2
  Mux7/1 -> RSC/3
  Mux2/1 -> RSC/5
  [idr1_ref] -> Mux2/1
  [idr1] -> Mux2/2
  [idr2] -> Mux2/4
  [idr2_ref] -> Mux2/3
  Mux8/1 -> RSC/6
  [vdr1_ref] -> Mux8/1
  [vqr2_ref] -> Mux8/2
  [vdg2_ref] -> Mux9/2
  Mux9/1 -> GSC/3
  [idg2_ref] -> Mux5/3
  [idg2] -> Mux5/4
  [iqg2_ref] -> Mux6/3
  [iqg2] -> Mux6/4
  [vqg2_ref] -> Mux10/2
  [vqg1_ref] -> Mux10/1
  Mux10/1 -> GSC/6

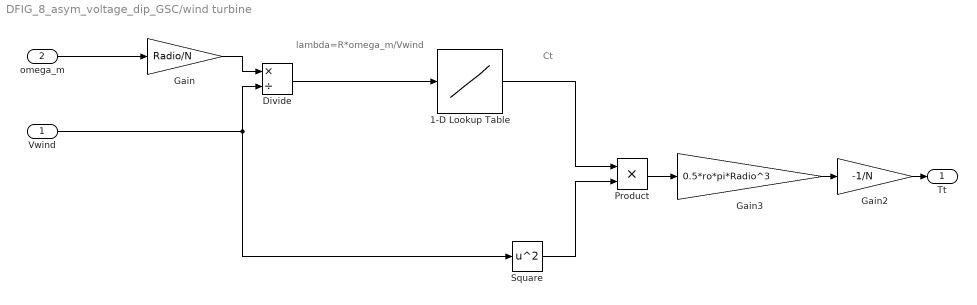
== system DFIG_8_asym_voltage_dip_GSC/wind turbine ==
  note: Ct
  note: lambda=R*omega_m/Vwind
  Vwind : Inport
  omega_m : Inport  Port=2
  1-D Lookup Table : Lookup_n-D  NumberOfTableDimensions=1  BreakpointsForDimension1=tab_lambda  Table=Ct  InternalRulePriority=Speed  RndMeth=Simplest
  Divide : Product  Inputs=*/
  Gain : Gain  Gain=Radio/N
  Gain2 : Gain  Gain=-1/N
  Gain3 : Gain  Gain=0.5*ro*pi*Radio^3
  Product : Product
  Square : Math  Operator=square
  Tt : Outport
  wires:
  Gain/1 -> Divide/1
  omega_m/1 -> Gain/1
  Vwind/1 -> Square/1, Divide/2
  Divide/1 -> 1-D Lookup Table/1
  Square/1 -> Product/2
  1-D Lookup Table/1 -> Product/1
  Product/1 -> Gain3/1
  Gain3/1 -> Gain2/1
  Gain2/1 -> Tt/1

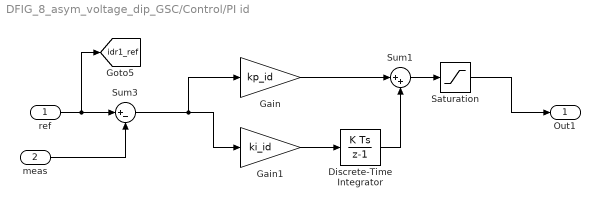
== system DFIG_8_asym_voltage_dip_GSC/Control/PI id ==
  ref : Inport
  meas : Inport  Port=2
  Discrete-Time Integrator : DiscreteIntegrator  SampleTime=1/fsw  LimitOutput=on  UpperSaturationLimit=Vbus/sqrt(3)  LowerSaturationLimit=-Vbus/sqrt(3)  ICPrevOutput=DiscIntNeverNeededParam  ICPrevScaledInput=DiscIntNeverNeededParam
  Gain : Gain  Gain=kp_id
  Gain1 : Gain  Gain=ki_id
  Saturation : Saturate  UpperLimit=Vbus/sqrt(3)  LowerLimit=-Vbus/sqrt(3)
  Sum1 : Sum  Inputs=|++
  Sum3 : Sum  Inputs=|+-
  Out1 : Outport
  tag scope: idr1_ref=global
  wires:
  meas/1 -> Sum3/2
  ref/1 -> [idr1_ref], Sum3/1
  Saturation/1 -> Out1/1
  Sum1/1 -> Saturation/1
  Discrete-Time Integrator/1 -> Sum1/2
  Gain/1 -> Sum1/1
  Gain1/1 -> Discrete-Time Integrator/1
  Sum3/1 -> Gain1/1, Gain/1

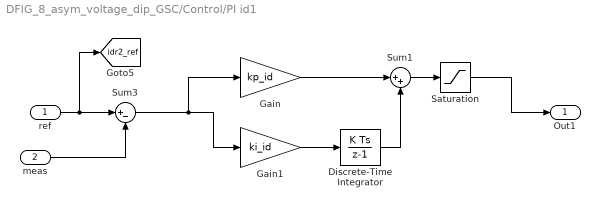
== system DFIG_8_asym_voltage_dip_GSC/Control/PI id1 ==
  ref : Inport
  meas : Inport  Port=2
  Discrete-Time Integrator : DiscreteIntegrator  SampleTime=1/fsw  LimitOutput=on  UpperSaturationLimit=Vbus/sqrt(3)  LowerSaturationLimit=-Vbus/sqrt(3)  ICPrevOutput=DiscIntNeverNeededParam  ICPrevScaledInput=DiscIntNeverNeededParam
  Gain : Gain  Gain=kp_id
  Gain1 : Gain  Gain=ki_id
  Saturation : Saturate  UpperLimit=Vbus/sqrt(3)  LowerLimit=-Vbus/sqrt(3)
  Sum1 : Sum  Inputs=|++
  Sum3 : Sum  Inputs=|+-
  Out1 : Outport
  tag scope: idr2_ref=global
  wires:
  Sum3/1 -> Gain/1, Gain1/1
  Gain1/1 -> Discrete-Time Integrator/1
  Gain/1 -> Sum1/1
  Discrete-Time Integrator/1 -> Sum1/2
  Sum1/1 -> Saturation/1
  Saturation/1 -> Out1/1
  ref/1 -> Sum3/1, [idr2_ref]
  meas/1 -> Sum3/2

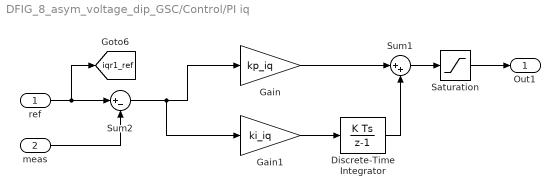
== system DFIG_8_asym_voltage_dip_GSC/Control/PI iq ==
  ref : Inport
  meas : Inport  Port=2
  Discrete-Time Integrator : DiscreteIntegrator  SampleTime=1/fsw  LimitOutput=on  UpperSaturationLimit=Vbus/sqrt(3)  LowerSaturationLimit=-Vbus/sqrt(3)  ICPrevOutput=DiscIntNeverNeededParam  ICPrevScaledInput=DiscIntNeverNeededParam
  Gain : Gain  Gain=kp_iq
  Gain1 : Gain  Gain=ki_iq
  Saturation : Saturate  UpperLimit=Vbus/sqrt(3)  LowerLimit=-Vbus/sqrt(3)
  Sum1 : Sum  Inputs=|++
  Sum2 : Sum  Inputs=|+-
  Out1 : Outport
  tag scope: iqr1_ref=global
  wires:
  ref/1 -> Sum2/1, [iqr1_ref]
  Saturation/1 -> Out1/1
  meas/1 -> Sum2/2
  Sum2/1 -> Gain/1, Gain1/1
  Gain1/1 -> Discrete-Time Integrator/1
  Gain/1 -> Sum1/1
  Discrete-Time Integrator/1 -> Sum1/2
  Sum1/1 -> Saturation/1

== system DFIG_8_asym_voltage_dip_GSC/Control/PI iq1 ==
  ref : Inport
  meas : Inport  Port=2
  Discrete-Time Integrator : DiscreteIntegrator  SampleTime=1/fsw  LimitOutput=on  UpperSaturationLimit=Vbus/sqrt(3)  LowerSaturationLimit=-Vbus/sqrt(3)  ICPrevOutput=DiscIntNeverNeededParam  ICPrevScaledInput=DiscIntNeverNeededParam
  Gain : Gain  Gain=kp_iq
  Gain1 : Gain  Gain=ki_iq
  Saturation : Saturate  UpperLimit=Vbus/sqrt(3)  LowerLimit=-Vbus/sqrt(3)
  Sum1 : Sum  Inputs=|++
  Sum2 : Sum  Inputs=|+-
  Out1 : Outport
  tag scope: iqr2_ref=global
  wires:
  Sum1/1 -> Saturation/1
  Discrete-Time Integrator/1 -> Sum1/2
  Gain/1 -> Sum1/1
  Gain1/1 -> Discrete-Time Integrator/1
  Sum2/1 -> Gain1/1, Gain/1
  meas/1 -> Sum2/2
  Saturation/1 -> Out1/1
  ref/1 -> [iqr2_ref], Sum2/1

== system DFIG_8_asym_voltage_dip_GSC/Control/PI speed ==
  in : Inport
  Discrete-Time Integrator : DiscreteIntegrator  SampleTime=1/fsw  LimitOutput=on  UpperSaturationLimit=Tem  LowerSaturationLimit=-Tem  ICPrevOutput=DiscIntNeverNeededParam  ICPrevScaledInput=DiscIntNeverNeededParam
  Gain : Gain  Gain=kp_n
  Gain1 : Gain  Gain=ki_n
  Saturation : Saturate  UpperLimit=Tem  LowerLimit=-Tem
  Sum1 : Sum  Inputs=|++
  Out : Outport
  wires:
  Saturation/1 -> Out/1
  Sum1/1 -> Saturation/1
  Discrete-Time Integrator/1 -> Sum1/2
  Gain/1 -> Sum1/1
  Gain1/1 -> Discrete-Time Integrator/1
  in/1 -> Gain/1, Gain1/1

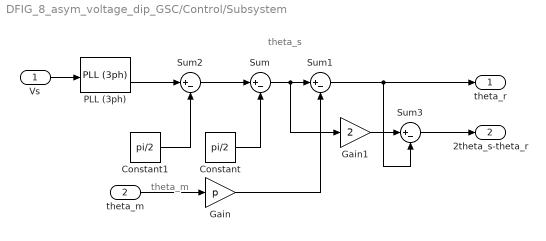
== system DFIG_8_asym_voltage_dip_GSC/Control/Subsystem ==
  note: theta_s
  note: theta_m
  Vs : Inport
  theta_m : Inport  Port=2
  Constant : Constant  Value=pi/2
  Constant1 : Constant  Value=pi/2
  Gain : Gain  Gain=p
  Gain1 : Gain  Gain=2
  PLL (3ph) : spsPLL3phLib/PLL (3ph)  Fmin=45  Par_Init=[0, 50]  ParK=[180, 3200, 1]  TcD=0.01  MaxRateChangeFreq=12  FilterCutOffFreq=25  Ts=1/fsw  AGC=on
  Sum{,1..3} (4 alike) : Sum  Inputs=|+-
  theta_r : Outport
  2theta_s-theta_r : Outport  Port=2
  wires:
  Vs/1 -> PLL (3ph)/1
  theta_m/1 -> Gain/1
  Sum2/1 -> Sum/1
  Constant/1 -> Sum/2
  Sum/1 -> Gain1/1, Sum1/1
  Sum1/1 -> Sum3/2, theta_r/1
  Gain/1 -> Sum1/2
  PLL (3ph)/2 -> Sum2/1
  Constant1/1 -> Sum2/2
  Sum3/1 -> 2theta_s-theta_r/1
  Gain1/1 -> Sum3/1

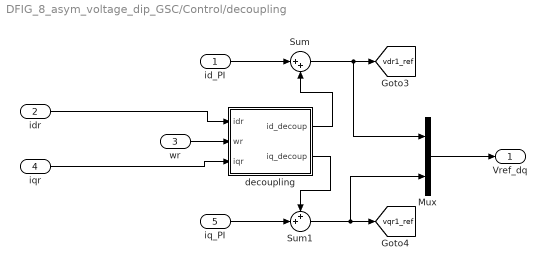
== system DFIG_8_asym_voltage_dip_GSC/Control/decoupling ==
  id_PI : Inport
  idr : Inport  Port=2
  wr : Inport  Port=3
  iqr : Inport  Port=4
  iq_PI : Inport  Port=5
  Mux : Mux  Inputs=2
  Sum : Sum  Inputs=|++
  Sum1 : Sum  Inputs=++|
  decoupling : Subsystem
  Vref_dq : Outport
  tag scope: vdr1_ref=global, vqr1_ref=global
  wires:
  decoupling/1(id_decoup) -> Sum/2
  Sum1/1 -> [vqr1_ref], Mux/2
  decoupling/2(iq_decoup) -> Sum1/1
  Sum/1 -> Mux/1, [vdr1_ref]
  wr/1 -> decoupling/2(wr)
  iq_PI/1 -> Sum1/2
  id_PI/1 -> Sum/1
  idr/1 -> decoupling/1(idr)
  Mux/1 -> Vref_dq/1
  iqr/1 -> decoupling/3(iqr)

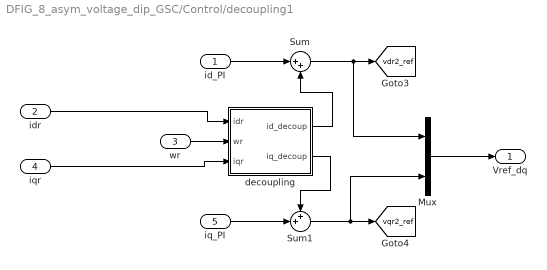
== system DFIG_8_asym_voltage_dip_GSC/Control/decoupling1 ==
  id_PI : Inport
  idr : Inport  Port=2
  wr : Inport  Port=3
  iqr : Inport  Port=4
  iq_PI : Inport  Port=5
  Mux : Mux  Inputs=2
  Sum : Sum  Inputs=|++
  Sum1 : Sum  Inputs=++|
  decoupling : Subsystem
  Vref_dq : Outport
  tag scope: vdr2_ref=global, vqr2_ref=global
  wires:
  iqr/1 -> decoupling/3(iqr)
  Mux/1 -> Vref_dq/1
  idr/1 -> decoupling/1(idr)
  id_PI/1 -> Sum/1
  iq_PI/1 -> Sum1/2
  wr/1 -> decoupling/2(wr)
  Sum/1 -> [vdr2_ref], Mux/1
  decoupling/2(iq_decoup) -> Sum1/1
  Sum1/1 -> Mux/2, [vqr2_ref]
  decoupling/1(id_decoup) -> Sum/2

== system DFIG_8_asym_voltage_dip_GSC/Control/harmonic injection ==
  abc : Inport
  Gain : Gain  Gain=-0.5
  Min : MinMax
  Min1 : MinMax  Function=max
  Sum : Sum  Inputs=|++
  Sum1 : Sum  Inputs=|++
  out : Outport
  wires:
  Min/1 -> Sum/1
  Min1/1 -> Sum/2
  Sum1/1 -> out/1
  Sum/1 -> Gain/1
  abc/1 -> Min1/1, Min/1, Sum1/1
  Gain/1 -> Sum1/2

== system DFIG_8_asym_voltage_dip_GSC/Control/indirect speed control ==
  omega_m : Inport
  Gain : Gain  Gain=1/N
  Gain1 : Gain  Gain=-Kopt
  Gain2 : Gain  Gain=1/N
  Square : Math  Operator=square
  Tem_ref : Outport
  wires:
  omega_m/1 -> Gain/1
  Gain/1 -> Square/1
  Gain2/1 -> Tem_ref/1
  Square/1 -> Gain1/1
  Gain1/1 -> Gain2/1

== system DFIG_8_asym_voltage_dip_GSC/Control1/PI Vbus ==
  in : Inport
  Discrete-Time Integrator : DiscreteIntegrator  SampleTime=1/fsw  LimitOutput=on  UpperSaturationLimit=Ps*smax  LowerSaturationLimit=-Ps*smax  ICPrevOutput=DiscIntNeverNeededParam  ICPrevScaledInput=DiscIntNeverNeededParam
  Gain : Gain  Gain=kp_v
  Gain1 : Gain  Gain=ki_v
  Saturation : Saturate  UpperLimit=Ps*smax  LowerLimit=-Ps*smax
  Sum1 : Sum  Inputs=|++
  Out : Outport
  wires:
  in/1 -> Gain1/1, Gain/1
  Gain1/1 -> Discrete-Time Integrator/1
  Gain/1 -> Sum1/1
  Discrete-Time Integrator/1 -> Sum1/2
  Sum1/1 -> Saturation/1
  Saturation/1 -> Out/1

== system DFIG_8_asym_voltage_dip_GSC/Control1/PI id ==
  in : Inport
  Discrete-Time Integrator : DiscreteIntegrator  SampleTime=1/fsw  LimitOutput=on  UpperSaturationLimit=Vbus*sqrt(3)  LowerSaturationLimit=-Vbus/sqrt(3)  ICPrevOutput=DiscIntNeverNeededParam  ICPrevScaledInput=DiscIntNeverNeededParam
  Gain : Gain  Gain=kp_idg
  Gain1 : Gain  Gain=ki_idg
  Saturation : Saturate  UpperLimit=Vbus/sqrt(3)  LowerLimit=-Vbus/sqrt(3)
  Sum1 : Sum  Inputs=|++
  Out : Outport
  wires:
  Saturation/1 -> Out/1
  Sum1/1 -> Saturation/1
  Discrete-Time Integrator/1 -> Sum1/2
  Gain/1 -> Sum1/1
  Gain1/1 -> Discrete-Time Integrator/1
  in/1 -> Gain/1, Gain1/1

== system DFIG_8_asym_voltage_dip_GSC/Control1/PI id1 ==
  in : Inport
  Discrete-Time Integrator : DiscreteIntegrator  SampleTime=1/fsw  LimitOutput=on  UpperSaturationLimit=Vbus*sqrt(3)  LowerSaturationLimit=-Vbus/sqrt(3)  ICPrevOutput=DiscIntNeverNeededParam  ICPrevScaledInput=DiscIntNeverNeededParam
  Gain : Gain  Gain=kp_idg
  Gain1 : Gain  Gain=ki_idg
  Saturation : Saturate  UpperLimit=Vbus/sqrt(3)  LowerLimit=-Vbus/sqrt(3)
  Sum1 : Sum  Inputs=|++
  Out : Outport
  wires:
  in/1 -> Gain1/1, Gain/1
  Gain1/1 -> Discrete-Time Integrator/1
  Gain/1 -> Sum1/1
  Discrete-Time Integrator/1 -> Sum1/2
  Sum1/1 -> Saturation/1
  Saturation/1 -> Out/1

== system DFIG_8_asym_voltage_dip_GSC/Control1/PI iq ==
  in : Inport
  Discrete-Time Integrator : DiscreteIntegrator  SampleTime=1/fsw  LimitOutput=on  UpperSaturationLimit=Vbus/sqrt(3)  LowerSaturationLimit=-Vbus/sqrt(3)  ICPrevOutput=DiscIntNeverNeededParam  ICPrevScaledInput=DiscIntNeverNeededParam
  Gain : Gain  Gain=kp_iqg
  Gain1 : Gain  Gain=ki_iqg
  Saturation : Saturate  UpperLimit=Vbus/sqrt(3)  LowerLimit=-Vbus/sqrt(3)
  Sum1 : Sum  Inputs=|++
  Out : Outport
  wires:
  in/1 -> Gain1/1, Gain/1
  Gain1/1 -> Discrete-Time Integrator/1
  Gain/1 -> Sum1/1
  Discrete-Time Integrator/1 -> Sum1/2
  Sum1/1 -> Saturation/1
  Saturation/1 -> Out/1

== system DFIG_8_asym_voltage_dip_GSC/Control1/PI iq1 ==
  in : Inport
  Discrete-Time Integrator : DiscreteIntegrator  SampleTime=1/fsw  LimitOutput=on  UpperSaturationLimit=Vbus/sqrt(3)  LowerSaturationLimit=-Vbus/sqrt(3)  ICPrevOutput=DiscIntNeverNeededParam  ICPrevScaledInput=DiscIntNeverNeededParam
  Gain : Gain  Gain=kp_iqg
  Gain1 : Gain  Gain=ki_iqg
  Saturation : Saturate  UpperLimit=Vbus/sqrt(3)  LowerLimit=-Vbus/sqrt(3)
  Sum1 : Sum  Inputs=|++
  Out : Outport
  wires:
  Saturation/1 -> Out/1
  Sum1/1 -> Saturation/1
  Discrete-Time Integrator/1 -> Sum1/2
  Gain/1 -> Sum1/1
  Gain1/1 -> Discrete-Time Integrator/1
  in/1 -> Gain/1, Gain1/1

== system DFIG_8_asym_voltage_dip_GSC/Control1/harmonic injection ==
  abc : Inport
  Gain : Gain  Gain=-0.5
  Min : MinMax
  Min1 : MinMax  Function=max
  Sum : Sum  Inputs=|++
  Sum1 : Sum  Inputs=|++
  out : Outport
  wires:
  Gain/1 -> Sum1/2
  abc/1 -> Sum1/1, Min/1, Min1/1
  Sum/1 -> Gain/1
  Sum1/1 -> out/1
  Min1/1 -> Sum/2
  Min/1 -> Sum/1

== system DFIG_8_asym_voltage_dip_GSC/Control/decoupling/decoupling ==
  note: -wr*sigma*Lr*iqr
  note: id decoupling
  note: iq decoupling
  idr : Inport
  wr : Inport  Port=2
  iqr : Inport  Port=3
  Gain3 : Gain  Gain=-sigma*Lr
  Gain4 : Gain  Gain=sigma*Lr
  Product : Product
  Product1 : Product
  id_decoup : Outport
  iq_decoup : Outport  Port=2
  wires:
  wr/1 -> Gain4/1, Gain3/1
  Product1/1 -> iq_decoup/1
  Gain3/1 -> Product/1
  Gain4/1 -> Product1/1
  iqr/1 -> Product/2
  idr/1 -> Product1/2
  Product/1 -> id_decoup/1

== system DFIG_8_asym_voltage_dip_GSC/Control/decoupling1/decoupling ==
  note: 负序控制器的解耦，符号和正序相反
  note: iq decoupling
  note: id decoupling
  idr : Inport
  wr : Inport  Port=2
  iqr : Inport  Port=3
  Gain3 : Gain  Gain=sigma*Lr
  Gain4 : Gain  Gain=-sigma*Lr
  Product : Product
  Product1 : Product
  id_decoup : Outport
  iq_decoup : Outport  Port=2
  wires:
  Product/1 -> id_decoup/1
  idr/1 -> Product1/2
  iqr/1 -> Product/2
  Gain4/1 -> Product1/1
  Gain3/1 -> Product/1
  Product1/1 -> iq_decoup/1
  wr/1 -> Gain3/1, Gain4/1

== matlab function DFIG_8_asym_voltage_dip_GSC/Control1/MATLAB Function7 ==
  data: ab0 input; abc output
function abc = ab0_to_abc(ab0)
abc = zeros(3,1);
abc(1) = ab0(1);
abc(2) = -1/2 * ab0(1) + sqrt(3)/2 * ab0(2);
abc(3) = -1/2 * ab0(1) - sqrt(3)/2 * ab0(2);
end

== matlab function DFIG_8_asym_voltage_dip_GSC/Control/MATLAB Function3 ==
  data: ab0 input; abc output
function abc = ab0_to_abc(ab0)
abc = zeros(3,1);
abc(1) = ab0(1);
abc(2) = -1/2 * ab0(1) + sqrt(3)/2 * ab0(2);
abc(3) = -1/2 * ab0(1) - sqrt(3)/2 * ab0(2);
end

== matlab function DFIG_8_asym_voltage_dip_GSC/Control/MATLAB Function4 ==
  data: dq input; ab0 output; theta input
function ab0 = dq_to_ab0(dq, theta)
ab0 = zeros(2,1);
ab0(1) = dq(1) * cos(theta) - dq(2) * sin(theta);
ab0(2) = dq(1) * sin(theta) + dq(2) * cos(theta);

end

== matlab function DFIG_8_asym_voltage_dip_GSC/Control/MATLAB Function2 ==
  data: ab0 input; dq output; theta input
function dq = ab0_to_dq(ab0, theta)
dq = zeros(2,1);
dq(1) = cos(theta)*ab0(1) + sin(theta)*ab0(2);
dq(2) = -sin(theta)*ab0(1) + cos(theta)*ab0(2);
end

== matlab function DFIG_8_asym_voltage_dip_GSC/Control1/MATLAB Function1 ==
  data: dq input; ab0 output; theta input
function ab0 = dq_to_ab0(dq, theta)
ab0 = zeros(2,1);
ab0(1) = dq(1) * cos(theta) - dq(2) * sin(theta);
ab0(2) = dq(1) * sin(theta) + dq(2) * cos(theta);

end

== matlab function DFIG_8_asym_voltage_dip_GSC/Control1/MATLAB Function2 ==
  data: ab0 input; dq output; theta input
function dq = ab0_to_dq(ab0, theta)
dq = zeros(2,1);
dq(1) = cos(theta)*ab0(1) + sin(theta)*ab0(2);
dq(2) = -sin(theta)*ab0(1) + cos(theta)*ab0(2);
end

== matlab function DFIG_8_asym_voltage_dip_GSC/Control1/MATLAB Function3 ==
  data: ab0 input; abc output
function abc = ab0_to_abc(ab0)
abc = zeros(3,1);
abc(1) = ab0(1);
abc(2) = -1/2 * ab0(1) + sqrt(3)/2 * ab0(2);
abc(3) = -1/2 * ab0(1) - sqrt(3)/2 * ab0(2);
end

== matlab function DFIG_8_asym_voltage_dip_GSC/Control/MATLAB Function6 ==
  data: abc input; ab0 output
function ab0 = abc_to_ab0(abc)
ab0 = zeros(2,1);
ab0(1) = 2/3 * (abc(1) - abc(2)/2 - abc(3)/2);
ab0(2) = 2/3 * ( (sqrt(3)/2)*abc(2) - (sqrt(3)/2)*abc(3));
end

== matlab function DFIG_8_asym_voltage_dip_GSC/Control1/MATLAB Function6 ==
  data: abc input; ab0 output
function ab0 = abc_to_ab0(abc)
ab0 = zeros(2,1);
ab0(1) = 2/3 * (abc(1) - abc(2)/2 - abc(3)/2);
ab0(2) = 2/3 * ( (sqrt(3)/2)*abc(2) - (sqrt(3)/2)*abc(3));
end

== matlab function DFIG_8_asym_voltage_dip_GSC/Control/MATLAB Function5 ==
  data: ab0 input; abc output
function abc = ab0_to_abc(ab0)
abc = zeros(3,1);
abc(1) = ab0(1);
abc(2) = -1/2 * ab0(1) + sqrt(3)/2 * ab0(2);
abc(3) = -1/2 * ab0(1) - sqrt(3)/2 * ab0(2);
end

== matlab function DFIG_8_asym_voltage_dip_GSC/Control/MATLAB Function1 ==
  data: dq input; ab0 output; theta input
function ab0 = dq_to_ab0(dq, theta)
ab0 = zeros(2,1);
ab0(1) = dq(1) * cos(theta) - dq(2) * sin(theta);
ab0(2) = dq(1) * sin(theta) + dq(2) * cos(theta);

end

== matlab function DFIG_8_asym_voltage_dip_GSC/Control1/MATLAB Function4 ==
  data: ab0 input; dq output; theta input
function dq = ab0_to_dq(ab0, theta)
dq = zeros(2,1);
dq(1) = cos(theta)*ab0(1) + sin(theta)*ab0(2);
dq(2) = -sin(theta)*ab0(1) + cos(theta)*ab0(2);
end

== matlab function DFIG_8_asym_voltage_dip_GSC/Control/MATLAB Function7 ==
  data: ab0 input; dq output; theta input
function dq = ab0_to_dq(ab0, theta)
dq = zeros(2,1);
dq(1) = cos(theta)*ab0(1) + sin(theta)*ab0(2);
dq(2) = -sin(theta)*ab0(1) + cos(theta)*ab0(2);
end

== matlab function DFIG_8_asym_voltage_dip_GSC/Control1/MATLAB Function5 ==
  data: dq input; ab0 output; theta input
function ab0 = dq_to_ab0(dq, theta)
ab0 = zeros(2,1);
ab0(1) = dq(1) * cos(theta) - dq(2) * sin(theta);
ab0(2) = dq(1) * sin(theta) + dq(2) * cos(theta);

end
